simulink model "simplexmodel"  (R2023a)
settings: Solver=FixedStepAuto  StartTime=0.0  StopTime=10.0  FixedStep=0.1  RelTol=1e-3
settings Model: Creator=rodri  LastModifiedBy=rodri

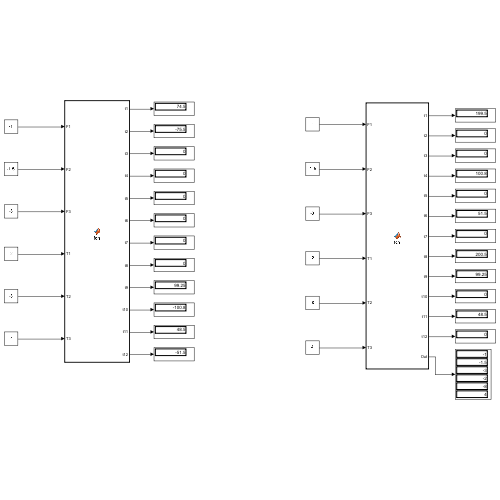
[thumbnail: Simulink's stored preview of the top-level diagram]
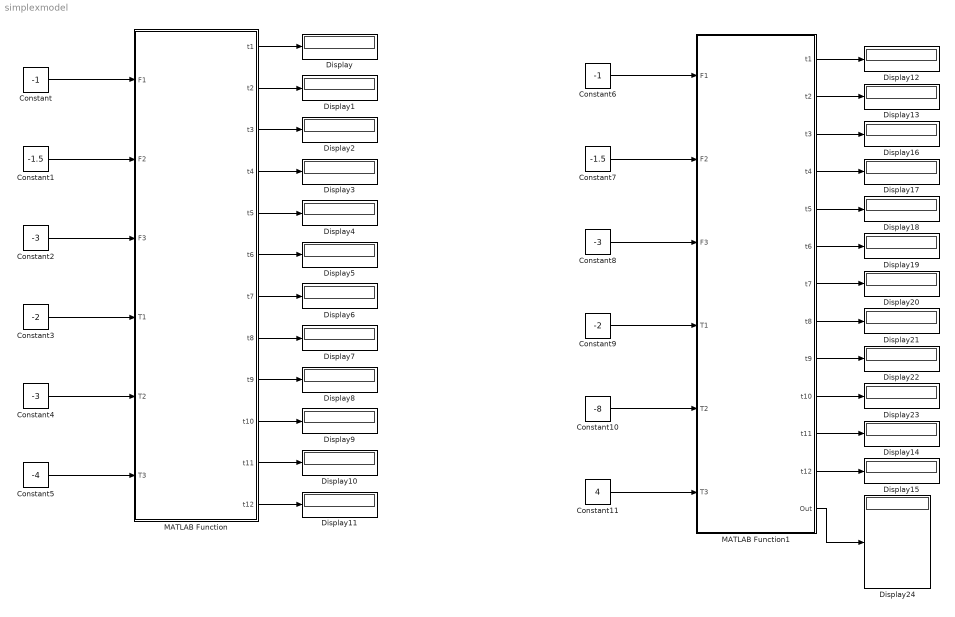
== system simplexmodel ==
  Constant : Constant  Value=-1
  Constant1 : Constant  Value=-1.5
  Constant10 : Constant  Value=-8
  Constant11 : Constant  Value=4
  Constant2 : Constant  Value=-3
  Constant3 : Constant  Value=-2
  Constant4 : Constant  Value=-3
  Constant5 : Constant  Value=-4
  Constant6 : Constant  Value=-1
  Constant7 : Constant  Value=-1.5
  Constant8 : Constant  Value=-3
  Constant9 : Constant  Value=-2
  Display{,1..24} (25 alike) : Display
  MATLAB Function : MATLAB Function  TreatAsAtomicUnit=on
  MATLAB Function1 : MATLAB Function  TreatAsAtomicUnit=on
  wires:
  MATLAB Function/1(t1) -> Display/1
  MATLAB Function/2(t2) -> Display1/1
  MATLAB Function/3(t3) -> Display2/1
  MATLAB Function/4(t4) -> Display3/1
  MATLAB Function/5(t5) -> Display4/1
  MATLAB Function/6(t6) -> Display5/1
  MATLAB Function/7(t7) -> Display6/1
  MATLAB Function/8(t8) -> Display7/1
  MATLAB Function/9(t9) -> Display8/1
  MATLAB Function/10(t10) -> Display9/1
  MATLAB Function/11(t11) -> Display10/1
  MATLAB Function/12(t12) -> Display11/1
  Constant5/1 -> MATLAB Function/6(T3)
  Constant4/1 -> MATLAB Function/5(T2)
  Constant3/1 -> MATLAB Function/4(T1)
  Constant/1 -> MATLAB Function/1(F1)
  Constant2/1 -> MATLAB Function/3(F3)
  Constant1/1 -> MATLAB Function/2(F2)
  Constant8/1 -> MATLAB Function1/3(F3)
  Constant7/1 -> MATLAB Function1/2(F2)
  Constant6/1 -> MATLAB Function1/1(F1)
  MATLAB Function1/7(t7) -> Display20/1
  MATLAB Function1/3(t3) -> Display16/1
  MATLAB Function1/10(t10) -> Display23/1
  MATLAB Function1/11(t11) -> Display14/1
  MATLAB Function1/4(t4) -> Display17/1
  MATLAB Function1/2(t2) -> Display13/1
  MATLAB Function1/6(t6) -> Display19/1
  MATLAB Function1/12(t12) -> Display15/1
  MATLAB Function1/9(t9) -> Display22/1
  MATLAB Function1/5(t5) -> Display18/1
  Constant10/1 -> MATLAB Function1/5(T2)
  MATLAB Function1/8(t8) -> Display21/1
  Constant9/1 -> MATLAB Function1/4(T1)
  Constant11/1 -> MATLAB Function1/6(T3)
  MATLAB Function1/1(t1) -> Display12/1
  MATLAB Function1/13(Out) -> Display24/1

== matlab function simplexmodel/MATLAB Function1 ==
  data: F1 input; t1 output; F2 input; F3 input; T1 input; T2 input; T3 input; t2 output; t3 output; t4 output; t5 output; t6 output; t7 output; t8 output; t9 output; t10 output; t11 output; t12 output; Out output
function [t1,t2,t3,t4,t5,t6,t7,t8,t9,t10,t11,t12,Out] = fcn(F1,F2,F3,T1,T2,T3)

F = [F1;F2;F3;T1;T2;T3];

Fn = 1;
Tn = Fn*2/100;

% A = [Fn Fn 0 0 0 0 -Fn -Fn 0 0 0 0
%     0 0 Fn Fn 0 0 0 0 -Fn -Fn 0 0
%     0 0 0 0 Fn Fn 0 0 0 0 -Fn -Fn
%     0 0 0 0 Tn -Tn 0 0 0 0 -Tn Tn
%     Tn -Tn 0 0 0 0 -Tn Tn 0 0 0 0
%     0 0 Tn -Tn 0 0 0 0 -Tn Tn 0 0];

A = [Fn Fn 0 0 0 0 -Fn -Fn 0 0 0 0
    0 0 -Fn -Fn 0 0 0 0 Fn Fn 0 0
    0 0 0 0 -Fn -Fn 0 0 0 0 Fn Fn
    0 0 0 0 Tn -Tn 0 0 0 0 -Tn Tn
    -Tn Tn 0 0 0 0 Tn -Tn 0 0 0 0
    0 0 -Tn Tn 0 0 0 0 Tn -Tn 0 0];

% if F(1)<0
%     A(1,:) = -A(1,:);
% elseif F(2)<0
%     A(2,:) = -A(2,:);
% elseif F(3)<0
%     A(3,:) = -A(3,:);
% elseif F(4)<0
%     A(4,:) = -A(4,:);
% elseif F(5)<0
%     A(5,:) = -A(5,:);
% elseif F(6)<0
%     A(6,:) = -A(6,:);
% end

c = [1 1 1 1 1 1 1 1 1 1 1 1];

[~,x] = nma_simplex(A,F,c,false);
%[~, ~, x, ~] = simplex('min', c, A, F);


t1 = x(1);
t2 = x(2);
t3 = x(3);
t4 = x(4);
t5 = x(5);
t6 = x(6);
t7 = x(7);
t8 = x(8);
t9 = x(9);
t10 = x(10);
t11 = x(11);
t12 = x(12);

if t1 < 0
    t7 = abs(t1);
    t1 = 0;
end

if t2 < 0
    t8 = abs(t2);
    t2 = 0;    
end

if t3 < 0
    t9 = abs(t3);
    t3 = 0;
end

if t4 < 0
    t10 = abs(t4);
    t4 = 0;
end

if t5 < 0
    t11 = abs(t5);
    t5 = 0;
end

if t6 < 0
    t12 = abs(t6);
    t6 = 0;
end

if t7 < 0
    t1 = abs(t7);
    t7 = 0;
end

if t8 < 0
    t2 = abs(t8);
    t8 = 0;
end

if t9 < 0
    t3 = abs(t9);
    t9 = 0;
end

if t10 < 0
    t4 = abs(t10);
    t10 = 0;
end

if t11 < 0
    t5 = abs(t11);
    t11 = 0;
end

if t12 < 0
    t6 = abs(t12);
    t12 = 0;
end

Out = A*[t1;t2;t3;t4;t5;t6;t7;t8;t9;t10;t11;t12];

== matlab function simplexmodel/MATLAB Function ==
  data: F1 input; t1 output; F2 input; F3 input; T1 input; T2 input; T3 input; t2 output; t3 output; t4 output; t5 output; t6 output; t7 output; t8 output; t9 output; t10 output; t11 output; t12 output
function [t1,t2,t3,t4,t5,t6,t7,t8,t9,t10,t11,t12] = fcn(F1,F2,F3,T1,T2,T3)

F = [F1;F2;F3;T1;T2;T3];

Fn = 1;
Tn = Fn*2/100;

% A = [Fn Fn 0 0 0 0 -Fn -Fn 0 0 0 0
%     0 0 Fn Fn 0 0 0 0 -Fn -Fn 0 0
%     0 0 0 0 Fn Fn 0 0 0 0 -Fn -Fn
%     0 0 0 0 Tn -Tn 0 0 0 0 -Tn Tn
%     Tn -Tn 0 0 0 0 -Tn Tn 0 0 0 0
%     0 0 Tn -Tn 0 0 0 0 -Tn Tn 0 0];

A = [Fn Fn 0 0 0 0 -Fn -Fn 0 0 0 0
    0 0 -Fn -Fn 0 0 0 0 Fn Fn 0 0
    0 0 0 0 -Fn -Fn 0 0 0 0 Fn Fn
    0 0 0 0 Tn -Tn 0 0 0 0 -Tn Tn
    -Tn Tn 0 0 0 0 Tn -Tn 0 0 0 0
    0 0 -Tn Tn 0 0 0 0 -Tn Tn 0 0];

% if F(1)<0
%     A(1,:) = -A(1,:);
% elseif F(2)<0
%     A(2,:) = -A(2,:);
% elseif F(3)<0
%     A(3,:) = -A(3,:);
% elseif F(4)<0
%     A(4,:) = -A(4,:);
% elseif F(5)<0
%     A(5,:) = -A(5,:);
% elseif F(6)<0
%     A(6,:) = -A(6,:);
% end

c = [1 1 1 1 1 1 1 1 1 1 1 1];

[~,x] = nma_simplex(A,F,c,false);
%[~, ~, x, ~] = simplex('min', c, A, F);


t1 = x(1);
t2 = x(2);
t3 = x(3);
t4 = x(4);
t5 = x(5);
t6 = x(6);
t7 = x(7);
t8 = x(8);
t9 = x(9);
t10 = x(10);
t11 = x(11);
t12 = x(12);
